simulink model "poblacion_sim"  (R2022b)
settings: Solver=VariableStepAuto  StartTime=0.0  StopTime=40.0  RelTol=1e-3
values from neighbouring files (symbols this model uses):
  initial_condition = 10    [poblacion.m]
  K = 0.0006    [poblacion.m]
  L = 500    [poblacion.m]
settings Model: Creator=Fran  LastModifiedBy=Fran

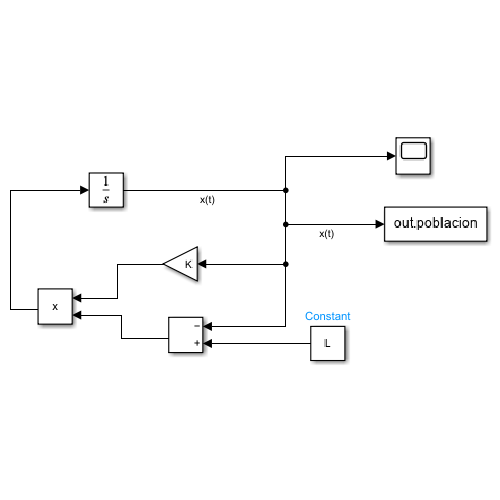
[thumbnail: Simulink's stored preview of the top-level diagram]
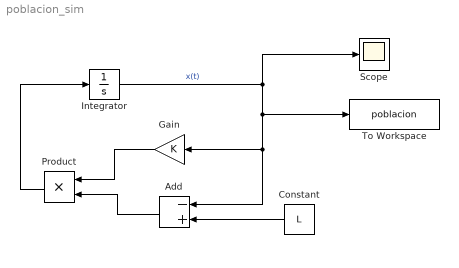
== system poblacion_sim ==
  Add : Sum  Inputs=-+
  Constant : Constant  Value=L
  Gain : Gain  Gain=K
  Integrator : Integrator  InitialCondition=initial_condition
  Product : Product
  Scope : Scope
  To Workspace : ToWorkspace  VariableName=poblacion  SampleTime=-1
  wires:
  Integrator/1 -> Scope/1, To Workspace/1, Add/1, Gain/1  "x(t)"
  Constant/1 -> Add/2
  Gain/1 -> Product/1
  Add/1 -> Product/2
  Product/1 -> Integrator/1
